simulink model "uas_demo"  (R2021a)
settings: Solver=FixedStepAuto  StartTime=0.0  StopTime=Inf  FixedStep=sample_time  RelTol=1e-3
model workspace: external: MAT-File (data not in the file)
values from neighbouring files (symbols this model uses):
  arm_length = 0.225    [Quadcopter_setup_parameters.m]    (also in recording.mat = 0.17; uas_parameters.m = 0.17; uas_parameters.mat = 0.17)
  drag_coefficient = 0.47    [Quadcopter_setup_parameters.m]    (also in recording.mat; uas_parameters.m; uas_parameters.mat)
  g = 9.81    [Quadcopter_setup_parameters.m]    (also in recording.mat = 9.80665; uas_parameters.m = 9.80665; uas_parameters.mat = 9.80665)
  inertia_xx = 5*10^(-3)    (= 0.005)    [Quadcopter_setup_parameters.m]    (also in recording.mat = 0.007; uas_parameters.m = 0.007; uas_parameters.mat = 0.007)
  inertia_yy = 5*10^(-3)    (= 0.005)    [Quadcopter_setup_parameters.m]    (also in recording.mat = 0.007; uas_parameters.m = 0.007; uas_parameters.mat = 0.007)
  inertia_zz = 8.9*10^(-3)    (= 0.0089)    [Quadcopter_setup_parameters.m]    (also in recording.mat = 0.012; uas_parameters.m = 0.012; uas_parameters.mat = 0.012)
  m = 0.55    [Quadcopter_setup_parameters.m]
  mass_drone = 0.55    [Quadcopter_setup_parameters.m]    (also in recording.mat = 0.68; uas_parameters.m = 0.68; uas_parameters.mat = 0.68)
  mass_total = mass_drone + mass_rod + mass_tip    (= 0.55)    [Quadcopter_setup_parameters.m]    (also in recording.mat = 0.68; uas_parameters.m = 0.68; uas_parameters.mat = 0.68)
  max_rot_velocity = 838    [Quadcopter_setup_parameters.m]    (also in recording.mat; uas_parameters.m; uas_parameters.mat)
  mix_matrix = inv(motor_constant * allocation_matrix)    [Quadcopter_setup_parameters.m]    (also in recording.mat = [29244.6230836 29244.6230836 29244.6230836 29244.6230836 -5.; uas_parameters.m; uas_parameters.mat = [29244.6230836 29244.6230836 29244.6230836 29244.6230836 -5.)
  moment_constant = 0.1    [Quadcopter_setup_parameters.m]    (also in recording.mat = 0.016; uas_parameters.m = 0.016; uas_parameters.mat = 0.016)
  motor_constant = 0.01    [Quadcopter_setup_parameters.m]    (also in recording.mat = 8.54858e-06; uas_parameters.m = 8.54858e-06; uas_parameters.mat = 8.54858e-06)
  p1 = 13.0908027334    [recording.mat]    (also in uas_parameters.mat = 12.1300541038; uas_thrust.mat = 12.1300541038; uas_thrust_constants.mat = 11.8019985126; uas_thrust_identification.m = result.p1)
  p2 = 0.438838137767    [recording.mat]    (also in uas_parameters.mat = 1.4832987942; uas_thrust.mat = 1.4832987942; uas_thrust_constants.mat = 1.1585190761; uas_thrust_identification.m = result.p2)
  poly_traj = PolyTrajGen(knots, order, optimization_target, dim, max_continuity)    [uas_minimum_snap.m]    (also in uas_trajectory.m = uas_minimum_snap(knots, order, waypoints, velocities, corrid)
  publish_rate = 1 * sample_time    (= 0.001)    [Quadcopter_setup_parameters.m]    (also in recording.mat = 0.04; uas_parameters.m = 0.04; uas_parameters.mat = 0.04)
  reference_area = pi * 75e-3^2    (= 0.0176714586764)    [Quadcopter_setup_parameters.m]    (also in recording.mat; uas_parameters.m; uas_parameters.mat)
  rotor_offset_top = 0.01    [Quadcopter_setup_parameters.m]    (also in recording.mat; uas_parameters.m; uas_parameters.mat)
  sample_time = 1e-3    (= 0.001)    [Quadcopter_setup_parameters.m]    (also in recording.mat = 0.04; uas_parameters.m = 0.04; uas_parameters.mat = 0.04)
  X = 3    [Quadcopter_setup_parameters.m]
  x0 = 36    [Quadcopter_setup_parameters.m]    (also in recording.mat; uas_parameters.m; uas_parameters.mat)
  Y = 2    [Quadcopter_setup_parameters.m]
  y0 = 80    [Quadcopter_setup_parameters.m]    (also in recording.mat; uas_parameters.m; uas_parameters.mat)
  Z = 1    [Quadcopter_setup_parameters.m]
  z0 = 1    [Quadcopter_setup_parameters.m]    (also in recording.mat = 0.3; uas_parameters.m; uas_parameters.mat)
undefined symbols (not defined in the file or in its folder): Angular, Linear, Pose, Position, Twist
libraries: nesl_utility x32, sm_lib x25, robotlib x13, simulink_extras x6, vrlib x1, sim3dlib x1, uavsim3dlib x1
(part 1 of 3)
settings Model: EnablePacing=on  Creator=david  LastModifiedBy=dwuth
settings SolverCC: AlgebraicLoopSolver=TrustRegion
settings DataIOCC: LimitDataPoints=on  MaxDataPoints=10000
settings OptimizationCC: EnhancedBackFolding=on  PassReuseOutputArgsThreshold=0  ZeroExternalMemoryAtStartup=off  ZeroInternalMemoryAtStartup=off  MaxStackSize=64  OptimizeBlockOrder=speed  DifferentSizesBufferReuse=on  OptimizationCustomize=off
settings DebuggingCC: ParameterTunabilityLossMsg=error  AllowSymbolicDim=off  SFUnexpectedBacktrackingDiag=warning  SFNoUnconditionalDefaultTransitionDiag=warning  SFExecutionAtInitializationDiag=none  SFMachineParentedDataDiag=warning  UnderSpecifiedDimensionMsg=warning  ArithmeticOperatorsInVariantConditions=warning
settings HardwareCC: ProdBitPerPointer=32  ProdBitPerSizeT=32  ProdBitPerPtrDiffT=32  ProdLargestAtomicFloat=None  ProdIntDivRoundTo=Undefined  ProdEndianess=Unspecified  ProdWordSize=32  ProdHWDeviceType=Generic->Unspecified (assume 32-bit Generic)  UseEmbeddedCoderFeatures=off
settings SFSimCC: SimUseLocalCustomCode=off  MATLABDynamicMemAlloc=off  CustomCodeUndefinedFunction=UseInterfaceOnly  SimTargetLang=C++
settings RTWCC: SystemTargetFile=ert.tlc  HardwareBoard=Robot Operating System (ROS)  TLCOptions="-aInlineSetEventsForThisBaseRateFcn=TLC_FALSE -aSuppressMultiTaskScheduler=TLC_FALSE  -aRateBasedStepFcn=0"  TemplateMakefile=ert_default_tmf  RTWUseLocalCustomCode=off  Toolchain=Catkin  TargetLang=C++
settings CodeAppCC: ForceParamTrailComments=on  OperatorAnnotations=on
settings ERTTargetCC: ERTCustomFileBanners=off  CodeInterfacePackaging=C++ class  SupportContinuousTime=on  SupportNonInlinedSFcns=on  RemoveResetFunc=off  ModelStepFunctionPrototypeControlCompliant=off  RootIOFormat=Structure reference
settings ConfigComp: CovMetricSettings=dw  CovSaveCumulativeToWorkspaceVar=on  CovSaveSingleToWorkspaceVar=on  CovExternalEMLEnable=off  CovSFcnEnable=off
settings SimscapeCC: SimscapeLogType=all  SimscapeLogSimulationStatistics=on  SimscapeLogDataHistory=10000

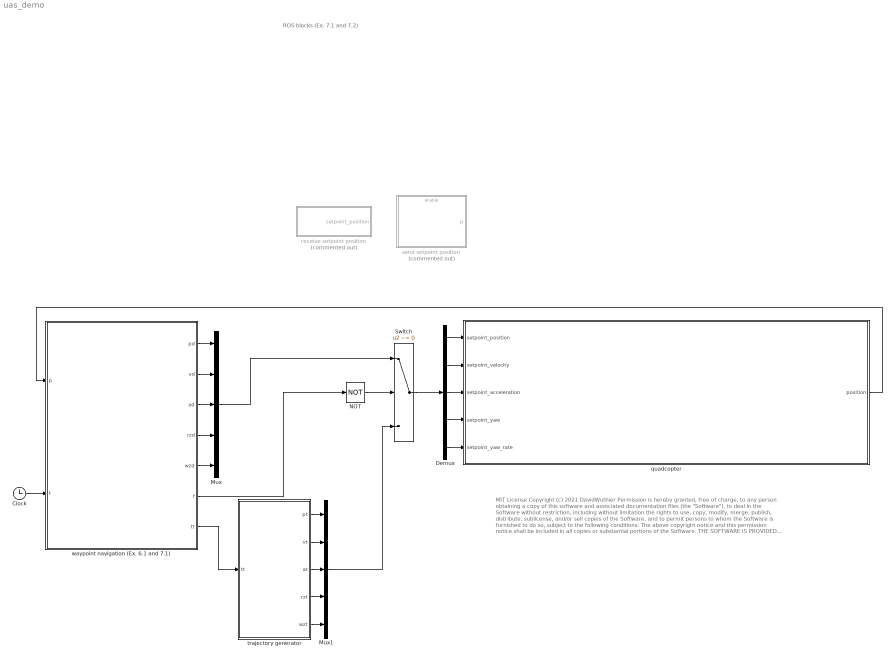
== system uas_demo ==
  note: MIT License
      |
      | Copyright (c) 2021 DavidWuthier
      |
      | Permission is hereby granted, free of charge, to any person obtaining a copy
      | of this software and associated documentation files (the "Software"), to deal
      | in the Software without restriction, including without limitation the rights
      | to use, copy, modify, merge, publish, distribute, sublicense, and/or sell
      | copies of the Software, and to permit persons to whom the Software is
      | furnished to do so, subject to the following conditions:
      |
      | The above copyright notice and this permission notice shall be included in all
      | copies or substantial portions of the Software.
      |
      | THE SOFTWARE IS PROVIDED "AS IS", WITHOUT WARRANTY OF ANY KIND, EXPRESS OR
      | IMPLIED, INCLUDING BUT NOT LIMITED TO THE WARRANTIES OF MERCHANTABILITY,
      | FITNESS FOR A PARTICULAR PURPOSE AND NONINFRINGEMENT. IN NO EVENT SHALL THE
      | AUTHORS OR COPYRIGHT HOLDERS BE LIABLE FOR ANY CLAIM, DAMAGES OR OTHER
      | LIABILITY, WHETHER IN AN ACTION OF CONTRACT, TORT OR OTHERWISE, ARISING FROM,
      | OUT OF OR IN CONNECTION WITH THE SOFTWARE OR THE USE OR OTHER DEALINGS IN THE
      | SOFTWARE.
  note: ROS blocks (Ex. 7.1 and 7.2)
  Clock : Clock
  Demux : Demux  Outputs=5
  Mux : Mux  Inputs=5
  Mux1 : Mux  Inputs=5
  NOT : Logic  Operator=NOT  IconShape=distinctive  AllPortsSameDT=off  OutDataTypeStr=boolean
  Switch : Switch  Criteria=u2 ~= 0
  quadcopter : Subsystem
  receive setpoint position : Subsystem  Commented=on
  send setpoint position : Subsystem  Commented=on
  trajectory generator : Subsystem
  waypoint navigation (Ex. 6.1 and 7.1) : Stateflow chart  TreatAsAtomicUnit=on
      settings: PortSchema="{\"entries\":[{\"content\":{\"sides\":[{\"content\":{\"connectorIds\":[\"In1\",\"In2\"]},\"type\":\"ConnectorPlacement.EquallySpacedRectSide\",\"uuid\":\"3b10aefc-58c0-4734-bcd6-9478d489aa11\"},{\"content\":{\"connectorIds\":[\"Out1\",\"Out2\",\"Out3\",\"Out7\",\"Out6\",\"Out5\",\"Out4\"],\"side\":\"RIGHT\"},\"type\":\"ConnectorPlacement.EquallySpacedRectSide\",\"uuid\":\"fcf7fbd2-2f8c-4d05-86e1-5a044196634d\"},{\"content\":{\"connectorIds\":[],\"side\":\"TOP\"},\"type\":\"ConnectorPlacement.EquallySpacedRectSide\",\"uuid\":\"94fc0c13-eb3b-4891-bff0-a1ef82a08378\"}]},\"type\":\"ConnectorPlacement.EquallySpacedConnector\",\"uuid\":\"15f9a3a1-5066-48dd-8188-11a3e0ea8b37\"}],\"packageUris\":[\"http://schema.mathworks.com/mf0/Connector/R2020b\"],\"version\":\"1.0\"}"
  wires:
  Clock/1 -> waypoint navigation (Ex. 6.1 and 7.1)/2(t)
  waypoint navigation (Ex. 6.1 and 7.1)/1(pd) -> Mux/1
  waypoint navigation (Ex. 6.1 and 7.1)/2(vd) -> Mux/2
  waypoint navigation (Ex. 6.1 and 7.1)/3(ad) -> Mux/3
  trajectory generator/1(pt) -> Mux1/1
  trajectory generator/2(vt) -> Mux1/2
  trajectory generator/3(at) -> Mux1/3
  waypoint navigation (Ex. 6.1 and 7.1)/4(tt) -> trajectory generator/1(tt)
  NOT/1 -> Switch/2
  waypoint navigation (Ex. 6.1 and 7.1)/5(f) -> NOT/1
  Mux1/1 -> Switch/3
  Mux/1 -> Switch/1
  Demux/1 -> quadcopter/1(setpoint_position)
  Demux/2 -> quadcopter/2(setpoint_velocity)
  Demux/3 -> quadcopter/3(setpoint_acceleration)
  Switch/1 -> Demux/1
  waypoint navigation (Ex. 6.1 and 7.1)/7(rzd) -> Mux/4
  waypoint navigation (Ex. 6.1 and 7.1)/6(wzd) -> Mux/5
  trajectory generator/4(rzt) -> Mux1/4
  trajectory generator/5(wzt) -> Mux1/5
  Demux/4 -> quadcopter/4(setpoint_yaw)
  Demux/5 -> quadcopter/5(setpoint_yaw_rate)
  quadcopter/1(position) -> waypoint navigation (Ex. 6.1 and 7.1)/1(p)

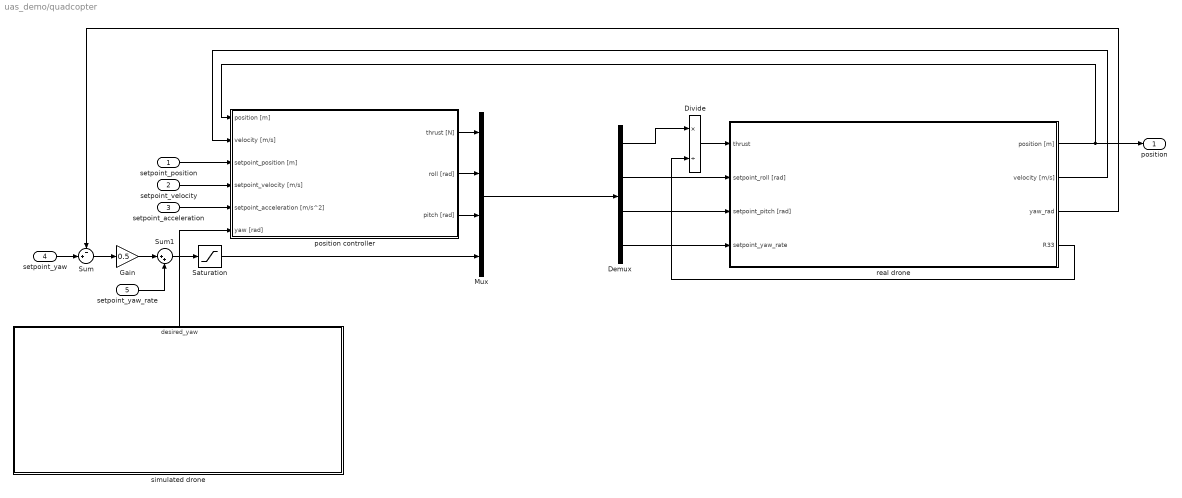
== system uas_demo/quadcopter ==
  setpoint_position : Inport  PortDimensions=[3 1]
  setpoint_velocity : Inport  Port=2  PortDimensions=[3 1]
  setpoint_acceleration : Inport  Port=3  PortDimensions=[3 1]
  setpoint_yaw : Inport  Port=4  PortDimensions=1
  setpoint_yaw_rate : Inport  Port=5  PortDimensions=1
  Demux : Demux
  Divide : Product  Inputs=*/
  Gain : Gain  Gain=0.5
  Mux : Mux
  Saturation : Saturate  UpperLimit=pi/2  LowerLimit=-pi/2
  Sum : Sum  Inputs=-+|
  Sum1 : Sum  Inputs=|++
  position controller : Subsystem
      mask Display: image('$imagefile'); % Use "Edit Image" on toolstrip to change.
  real drone : Subsystem
  simulated drone : Subsystem
      settings: PortSchema="{\"entries\":[{\"content\":{\"sides\":[{\"content\":{\"connectorIds\":[]},\"type\":\"ConnectorPlacement.EquallySpacedRectSide\",\"uuid\":\"a4b6e2c3-de70-4302-a56e-c646c409cb1c\"},{\"content\":{\"connectorIds\":[],\"side\":\"RIGHT\"},\"type\":\"ConnectorPlacement.EquallySpacedRectSide\",\"uuid\":\"cf331e27-abc1-4524-81a0-eea9b20dbeff\"},{\"content\":{\"connectorIds\":[\"Out1\"],\"side\":\"TOP\"},\"type\":\"ConnectorPlacement.EquallySpacedRectSide\",\"uuid\":\"8fd6f6ce-4f1c-4c94-a1c8-f1d72f1bbfd5\"},{\"content\":{\"connectorIds\":[],\"side\":\"BOTTOM\"},\"type\":\"ConnectorPlacement.EquallySpacedRectSide\",\"uuid\":\"db19f303-95c2-42a9-9683-bd7cccf66e90\"}]},\"type\":\"ConnectorPlacement.EquallySpacedConnector\",\"uuid\":\"27e9fd01-12c5-44cf-b1f4-f7b3cd5ad227\"}],\"packageUris\":[\"http://schema.mathworks.com/mf0/Connector/R2020b\"],\"version\":\"1.0\"}"
  position : Outport
  wires:
  setpoint_acceleration/1 -> position controller/5(setpoint_acceleration [m/s^2])
  setpoint_velocity/1 -> position controller/4(setpoint_velocity [m/s])
  setpoint_position/1 -> position controller/3(setpoint_position [m])
  position controller/1(thrust [N]) -> Mux/1
  position controller/2(roll [rad]) -> Mux/2
  position controller/3(pitch [rad]) -> Mux/3
  Demux/1 -> Divide/1
  Sum/1 -> Gain/1
  setpoint_yaw/1 -> Sum/2
  Gain/1 -> Sum1/1
  setpoint_yaw_rate/1 -> Sum1/2
  Sum1/1 -> Saturation/1
  Saturation/1 -> Mux/4
  real drone/1(position [m]) -> position/1, position controller/1(position [m])
  Divide/1 -> real drone/1(thrust)
  Demux/2 -> real drone/2(setpoint_roll [rad])
  Demux/3 -> real drone/3(setpoint_pitch [rad])
  Demux/4 -> real drone/4(setpoint_yaw_rate)
  real drone/2(velocity [m/s]) -> position controller/2(velocity [m/s])
  real drone/3(yaw_rad) -> Sum/1
  Mux/1 -> Demux/1
  simulated drone/1(desired_yaw) -> position controller/6(yaw [rad])
  real drone/4(R33) -> Divide/2

== system uas_demo/receive setpoint position ==
  Bus Selector : BusSelector  OutputSignals=Position.X,Position.Y,Position.Z
  Mux : Mux  Inputs=3
  Subscribe : robotlib/Subscribe  topicSource=Specify your own  topic=/crazyflie/cmd_position  messageType=geometry_msgs/Pose  SampleTime=-1  legacyBusStruct=off  messageQueueLength=1
  Terminator5 : Terminator
  setpoint_position : Outport
  wires:
  Subscribe/2 -> Bus Selector/1
  Mux/1 -> setpoint_position/1
  Bus Selector/3 -> Mux/3  "<Z>"
  Bus Selector/1 -> Mux/1  "<X>"
  Bus Selector/2 -> Mux/2  "<Y>"
  Subscribe/1 -> Terminator5/1

== system uas_demo/send setpoint position ==
  p : Inport
  Enable : EnablePort
  send setpoint position : Subsystem
  wires:
  p/1 -> send setpoint position/1(p)

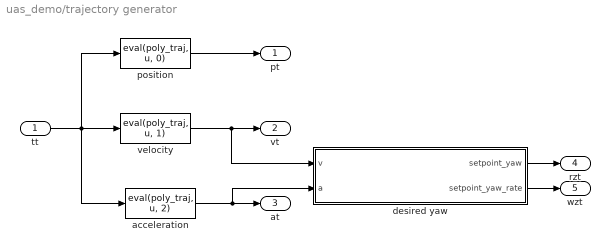
== system uas_demo/trajectory generator ==
  tt : Inport
  acceleration : MATLABFcn  MATLABFcn=eval(poly_traj, u, 2)  OutputDimensions=[3 1]  Output1D=off
  desired yaw : MATLAB Function  TreatAsAtomicUnit=on
  position : MATLABFcn  MATLABFcn=eval(poly_traj, u, 0)  OutputDimensions=[3 1]  Output1D=off
  velocity : MATLABFcn  MATLABFcn=eval(poly_traj, u, 1)  OutputDimensions=[3 1]  Output1D=off
  pt : Outport
  vt : Outport  Port=2
  at : Outport  Port=3
  rzt : Outport  Port=4
  wzt : Outport  Port=5
  wires:
  tt/1 -> acceleration/1, position/1, velocity/1
  velocity/1 -> desired yaw/1(v), vt/1
  position/1 -> pt/1
  acceleration/1 -> desired yaw/2(a), at/1
  desired yaw/1(setpoint_yaw) -> rzt/1
  desired yaw/2(setpoint_yaw_rate) -> wzt/1

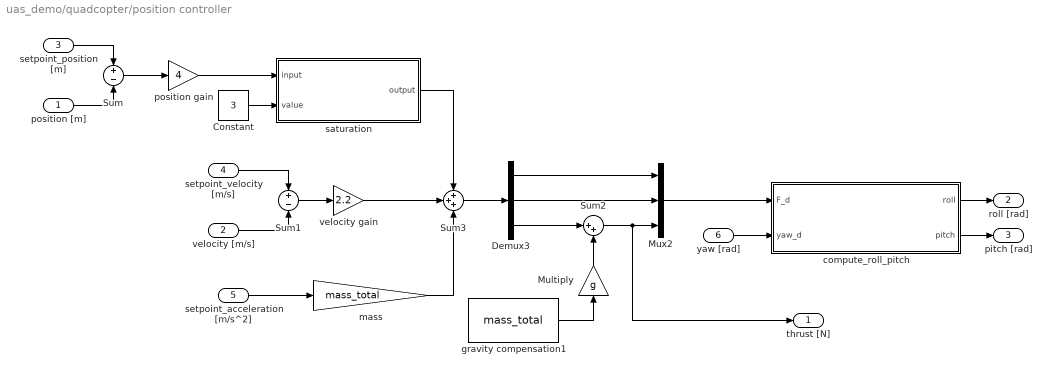
== system uas_demo/quadcopter/position controller ==
  position [m] : Inport
  velocity [m/s] : Inport  Port=2
  setpoint_position [m] : Inport  Port=3
  setpoint_velocity [m/s] : Inport  Port=4
  setpoint_acceleration [m/s^2] : Inport  Port=5
  yaw [rad] : Inport  Port=6
  Constant : Constant  Value=3
  Demux3 : Demux  Outputs=3
  Multiply : Gain  Gain=g
  Mux2 : Mux  Inputs=3
  Sum : Sum  Inputs=+|-
  Sum1 : Sum  Inputs=+|-
  Sum2 : Sum  Inputs=|++
  Sum3 : Sum  Inputs=+++
  compute_roll_pitch : MATLAB Function  TreatAsAtomicUnit=on
  gravity compensation1 : Constant  Value=mass_total  VectorParams1D=off
  mass : Gain  Gain=mass_total
  position gain : Gain  Gain=4
  saturation : Subsystem
  velocity gain : Gain  Gain=2.2
  thrust [N] : Outport
  roll [rad] : Outport  Port=2
  pitch [rad] : Outport  Port=3
  wires:
  saturation/1(output) -> Sum3/1
  position gain/1 -> saturation/1(input)
  gravity compensation1/1 -> Multiply/1
  velocity [m/s]/1 -> Sum1/2
  Demux3/3 -> Sum2/1
  mass/1 -> Sum3/3
  Constant/1 -> saturation/2(value)
  Sum2/1 -> thrust [N]/1, Mux2/3
  Sum1/1 -> velocity gain/1
  velocity gain/1 -> Sum3/2
  Sum/1 -> position gain/1
  Sum3/1 -> Demux3/1
  Demux3/1 -> Mux2/1
  Mux2/1 -> compute_roll_pitch/1(F_d)
  Demux3/2 -> Mux2/2
  compute_roll_pitch/1(roll) -> roll [rad]/1
  Multiply/1 -> Sum2/2
  setpoint_position [m]/1 -> Sum/1
  compute_roll_pitch/2(pitch) -> pitch [rad]/1
  position [m]/1 -> Sum/2
  yaw [rad]/1 -> compute_roll_pitch/2(yaw_d)
  setpoint_velocity [m/s]/1 -> Sum1/1
  setpoint_acceleration [m/s^2]/1 -> mass/1

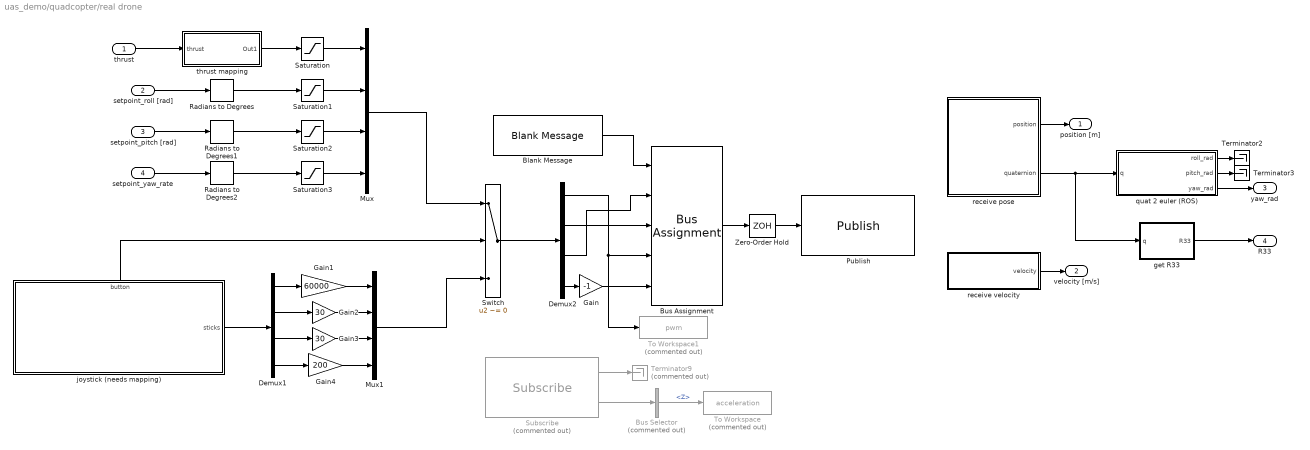
== system uas_demo/quadcopter/real drone ==
  thrust : Inport
  setpoint_roll [rad] : Inport  Port=2
  setpoint_pitch [rad] : Inport  Port=3
  setpoint_yaw_rate : Inport  Port=4
  Blank Message : robotlib/Blank Message  messageClass=Message  entityType=geometry_msgs/Twist  messageType=geometry_msgs/Twist  SampleTime=inf  legacyBusStruct=off
  Bus Assignment : BusAssignment  AssignedSignals=Linear.X,Linear.Y,Linear.Z,Angular.Z
  Bus Selector : BusSelector  Commented=on  OutputSignals=LinearAcceleration.Z
  Demux1 : Demux
  Demux2 : Demux
  Gain : Gain  Gain=-1
  Gain1 : Gain  Gain=60000
  Gain2 : Gain  Gain=30
  Gain3 : Gain  Gain=30
  Gain4 : Gain  Gain=200
  Mux : Mux
  Mux1 : Mux
  Publish : robotlib/Publish  topicSource=Select from ROS network  topic=/crazyflie/cmd_vel  messageType=geometry_msgs/Twist  legacyBusStruct=off  messageQueueLength=1
  Radians to Degrees : simulink_extras/Transformations/Radians to Degrees
  Radians to Degrees1 : simulink_extras/Transformations/Radians to Degrees
  Radians to Degrees2 : simulink_extras/Transformations/Radians to Degrees
  Saturation : Saturate  UpperLimit=50000  LowerLimit=5000
  Saturation1 : Saturate  UpperLimit=10  LowerLimit=-10
  Saturation2 : Saturate  UpperLimit=10  LowerLimit=-10
  Saturation3 : Saturate  UpperLimit=90  LowerLimit=-90
  Subscribe : robotlib/Subscribe  Commented=on  topicSource=Select from ROS network  topic=/crazyflie/imu  messageType=sensor_msgs/Imu  SampleTime=-1  legacyBusStruct=off  messageQueueLength=1
  Switch : Switch  Criteria=u2 ~= 0
  Terminator2 : Terminator
  Terminator3 : Terminator
  Terminator9 : Terminator  Commented=on
  To Workspace : ToWorkspace  Commented=on  VariableName=acceleration  SaveFormat=Timeseries  SampleTime=-1
  To Workspace1 : ToWorkspace  Commented=on  VariableName=pwm  SaveFormat=Timeseries  SampleTime=-1
  Zero-Order Hold : ZeroOrderHold  SampleTime=1/25
  get R33 : MATLAB Function  TreatAsAtomicUnit=on
  joystick (needs mapping) : Subsystem
      settings: PortSchema="{\"entries\":[{\"content\":{\"sides\":[{\"content\":{\"connectorIds\":[]},\"type\":\"ConnectorPlacement.EquallySpacedRectSide\",\"uuid\":\"5fda1310-e934-4f88-a5ae-12eb429239ff\"},{\"content\":{\"connectorIds\":[\"Out1\"],\"side\":\"RIGHT\"},\"type\":\"ConnectorPlacement.EquallySpacedRectSide\",\"uuid\":\"2a21e2c7-e332-4e9d-ba4f-bafdc6371a4a\"},{\"content\":{\"connectorIds\":[\"Out2\"],\"side\":\"TOP\"},\"type\":\"ConnectorPlacement.EquallySpacedRectSide\",\"uuid\":\"ad915a58-fa45-4be6-9ede-fc828b040a89\"}]},\"type\":\"ConnectorPlacement.EquallySpacedConnector\",\"uuid\":\"284bbdda-bb32-4fe9-aff6-c2c88357457c\"}],\"packageUris\":[\"http://schema.mathworks.com/mf0/Connector/R2020b\"],\"version\":\"1.0\"}"
  quat 2 euler (ROS) : MATLAB Function  TreatAsAtomicUnit=on
  receive pose : Subsystem
      settings: PortSchema="{\"entries\":[{\"content\":{\"sides\":[{\"content\":{\"connectorIds\":[\"Out1\",\"Out2\"]},\"type\":\"ConnectorPlacement.EquallySpacedRectSide\",\"uuid\":\"342eff32-bd5e-4bb8-a2c1-1476062da077\"},{\"content\":{\"connectorIds\":[],\"side\":\"RIGHT\"},\"type\":\"ConnectorPlacement.EquallySpacedRectSide\",\"uuid\":\"5f12c17c-6870-4adf-b6d3-8aed3aa982af\"},{\"content\":{\"connectorIds\":[],\"side\":\"TOP\"},\"type\":\"ConnectorPlacement.EquallySpacedRectSide\",\"uuid\":\"ee216cdd-c6bd-4d8d-9854-9a410974daca\"}]},\"type\":\"ConnectorPlacement.EquallySpacedConnector\",\"uuid\":\"aa6eedf3-0c3b-49f1-8a80-dfaeacb28973\"}],\"packageUris\":[\"http://schema.mathworks.com/mf0/Connector/R2020b\"],\"version\":\"1.0\"}"
  receive velocity : Subsystem
      settings: PortSchema="{\"entries\":[{\"content\":{\"sides\":[{\"content\":{\"connectorIds\":[\"Out1\"]},\"type\":\"ConnectorPlacement.EquallySpacedRectSide\",\"uuid\":\"342eff32-bd5e-4bb8-a2c1-1476062da077\"},{\"content\":{\"connectorIds\":[],\"side\":\"RIGHT\"},\"type\":\"ConnectorPlacement.EquallySpacedRectSide\",\"uuid\":\"5f12c17c-6870-4adf-b6d3-8aed3aa982af\"},{\"content\":{\"connectorIds\":[],\"side\":\"TOP\"},\"type\":\"ConnectorPlacement.EquallySpacedRectSide\",\"uuid\":\"ee216cdd-c6bd-4d8d-9854-9a410974daca\"}]},\"type\":\"ConnectorPlacement.EquallySpacedConnector\",\"uuid\":\"aa6eedf3-0c3b-49f1-8a80-dfaeacb28973\"}],\"packageUris\":[\"http://schema.mathworks.com/mf0/Connector/R2020b\"],\"version\":\"1.0\"}"
  thrust mapping : Subsystem
  position [m] : Outport
  velocity [m/s] : Outport  Port=2
  yaw_rad : Outport  Port=3
  R33 : Outport  Port=4
  wires:
  quat 2 euler (ROS)/2(pitch_rad) -> Terminator3/1
  quat 2 euler (ROS)/3(yaw_rad) -> yaw_rad/1
  quat 2 euler (ROS)/1(roll_rad) -> Terminator2/1
  receive pose/1(position) -> position [m]/1
  receive velocity/1(velocity) -> velocity [m/s]/1
  receive pose/2(quaternion) -> get R33/1(q), quat 2 euler (ROS)/1(q)
  thrust/1 -> thrust mapping/1(thrust)
  setpoint_roll [rad]/1 -> Radians to Degrees/1
  setpoint_pitch [rad]/1 -> Radians to Degrees1/1
  setpoint_yaw_rate/1 -> Radians to Degrees2/1
  Zero-Order Hold/1 -> Publish/1
  Demux2/3 -> Bus Assignment/2
  Demux2/4 -> Gain/1
  Blank Message/1 -> Bus Assignment/1
  Bus Assignment/1 -> Zero-Order Hold/1
  Demux2/2 -> Bus Assignment/3
  Demux2/1 -> To Workspace1/1, Bus Assignment/4
  Radians to Degrees/1 -> Saturation1/1
  Radians to Degrees1/1 -> Saturation2/1
  Radians to Degrees2/1 -> Saturation3/1
  Saturation1/1 -> Mux/2
  Saturation2/1 -> Mux/3
  Saturation3/1 -> Mux/4
  Saturation/1 -> Mux/1
  Switch/1 -> Demux2/1
  Mux/1 -> Switch/1
  Gain3/1 -> Mux1/3
  Gain2/1 -> Mux1/2
  Demux1/2 -> Gain2/1
  Demux1/3 -> Gain3/1
  Demux1/4 -> Gain4/1
  Demux1/1 -> Gain1/1
  Gain4/1 -> Mux1/4
  Gain1/1 -> Mux1/1
  joystick (needs mapping)/1(sticks) -> Demux1/1
  Mux1/1 -> Switch/3
  joystick (needs mapping)/2(button) -> Switch/2
  Bus Selector/1 -> To Workspace/1  "<Z>"
  Subscribe/1 -> Terminator9/1
  Subscribe/2 -> Bus Selector/1
  thrust mapping/1(Out1) -> Saturation/1
  Gain/1 -> Bus Assignment/5
  get R33/1(R33) -> R33/1

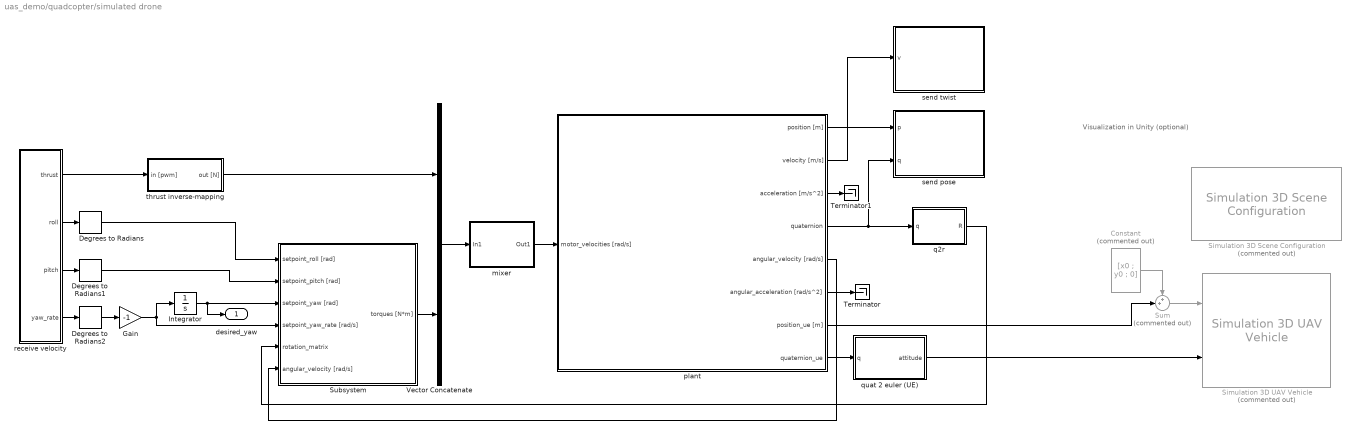
== system uas_demo/quadcopter/simulated drone ==
  note: Visualization in Unity (optional)
  Constant : Constant  Commented=on  Value=[x0 ; y0 ; 0]  VectorParams1D=off
  Degrees to Radians : simulink_extras/Transformations/Degrees to Radians
  Degrees to Radians1 : simulink_extras/Transformations/Degrees to Radians
  Degrees to Radians2 : simulink_extras/Transformations/Degrees to Radians
  Gain : Gain  Gain=-1
  Integrator : Integrator  WrapState=on
  Simulation 3D Scene Configuration : sim3dlib/Simulation 3D Scene Configuration  Priority=0  Commented=on  ProjectFormat=Default Scenes  SceneDesc=US city block  ProjectName=C:\Program Files\MATLAB\R2021a\toolbox\shared\sim3d_projects\automotive_project\UE4\WindowsNoEditor\VehicleSimulation.exe  ScenePath=/Game/Maps/USCityBlock  vehTagList={'Scene Origin';'SimulinkVehicle1'}  vehTag=SimulinkVehicle1  OpVisEn=off  Ts=sample_time  EnableWindow=on  EnableWeather=off  SunAltitude=40.0  SunAzimuth=90  clouds=10  wind=1  fog=0  rain=0  sensorTag=MainCamera1  sensorId=1  sensorName=MainCamera1  mountLoc=Origin  offsetFlag=off  tmountOffset=[0, 0, 0]  rmountOffset=[0, 0, 0]  HorizontalResolution=1280  VerticalResolution=720  HorizontalFOV=60  mountPoint=[0 0 0]  mountOrientation=[0 0 0]  aMode=4  ID=1
      settings: SourceProductBaseCode=DR,UV,VE
  Simulation 3D UAV Vehicle : uavsim3dlib/Simulation 3D UAV Vehicle  Commented=on  Mesh=Quadrotor  Color=Green  ActorName=SimulinkVehicle1  InitialTranslation=[x0 y0 z0]  InitialRotation=[0 0 0]  SampleTime=-1  ActorType=SimulinkVehicle  ID=1  aMode=4  ActorTag=SimulinkVehicle1
      settings: SourceProductBaseCode=UV
  Subsystem : Subsystem
      mask Display: image('$imagefile'); % Use "Edit Image" on toolstrip to change.
  Sum : Sum  Commented=on  Inputs=++|
  Terminator : Terminator
  Terminator1 : Terminator
  Vector Concatenate : Concatenate
  mixer : Subsystem
  plant : Subsystem
      mask Display: image('$imagefile'); % Use "Edit Image" on toolstrip to change.
  q2r : MATLAB Function  TreatAsAtomicUnit=on
  quat 2 euler (UE) : MATLAB Function  TreatAsAtomicUnit=on
  receive velocity : Subsystem
      settings: PortSchema="{\"entries\":[{\"content\":{\"sides\":[{\"content\":{\"connectorIds\":[\"Out1\",\"Out2\",\"Out3\",\"Out4\"]},\"type\":\"ConnectorPlacement.EquallySpacedRectSide\",\"uuid\":\"342eff32-bd5e-4bb8-a2c1-1476062da077\"},{\"content\":{\"connectorIds\":[],\"side\":\"RIGHT\"},\"type\":\"ConnectorPlacement.EquallySpacedRectSide\",\"uuid\":\"5f12c17c-6870-4adf-b6d3-8aed3aa982af\"},{\"content\":{\"connectorIds\":[],\"side\":\"TOP\"},\"type\":\"ConnectorPlacement.EquallySpacedRectSide\",\"uuid\":\"ee216cdd-c6bd-4d8d-9854-9a410974daca\"}]},\"type\":\"ConnectorPlacement.EquallySpacedConnector\",\"uuid\":\"aa6eedf3-0c3b-49f1-8a80-dfaeacb28973\"}],\"packageUris\":[\"http://schema.mathworks.com/mf0/Connector/R2020b\"],\"version\":\"1.0\"}"
  send pose : Subsystem
      settings: PortSchema="{\"entries\":[{\"content\":{\"sides\":[{\"content\":{\"connectorIds\":[]},\"type\":\"ConnectorPlacement.EquallySpacedRectSide\",\"uuid\":\"91ac49ce-0d45-467e-8a0f-3e047764dac5\"},{\"content\":{\"connectorIds\":[\"In1\",\"In2\"],\"side\":\"RIGHT\"},\"type\":\"ConnectorPlacement.EquallySpacedRectSide\",\"uuid\":\"1d243291-4bc7-414c-85ed-69dd8ac9cef1\"},{\"content\":{\"connectorIds\":[],\"side\":\"TOP\"},\"type\":\"ConnectorPlacement.EquallySpacedRectSide\",\"uuid\":\"579f94ca-36dc-4d39-8b83-523f53ee323c\"}]},\"type\":\"ConnectorPlacement.EquallySpacedConnector\",\"uuid\":\"95d78beb-d4cc-4232-87a4-7f0d7b157e3f\"}],\"packageUris\":[\"http://schema.mathworks.com/mf0/Connector/R2020b\"],\"version\":\"1.0\"}"
  send twist : Subsystem
      settings: PortSchema="{\"entries\":[{\"content\":{\"sides\":[{\"content\":{\"connectorIds\":[]},\"type\":\"ConnectorPlacement.EquallySpacedRectSide\",\"uuid\":\"91ac49ce-0d45-467e-8a0f-3e047764dac5\"},{\"content\":{\"connectorIds\":[\"In1\"],\"side\":\"RIGHT\"},\"type\":\"ConnectorPlacement.EquallySpacedRectSide\",\"uuid\":\"1d243291-4bc7-414c-85ed-69dd8ac9cef1\"},{\"content\":{\"connectorIds\":[],\"side\":\"TOP\"},\"type\":\"ConnectorPlacement.EquallySpacedRectSide\",\"uuid\":\"579f94ca-36dc-4d39-8b83-523f53ee323c\"}]},\"type\":\"ConnectorPlacement.EquallySpacedConnector\",\"uuid\":\"95d78beb-d4cc-4232-87a4-7f0d7b157e3f\"}],\"packageUris\":[\"http://schema.mathworks.com/mf0/Connector/R2020b\"],\"version\":\"1.0\"}"
  thrust inverse-mapping : Subsystem
  desired_yaw : Outport
  wires:
  quat 2 euler (UE)/1(attitude) -> Simulation 3D UAV Vehicle/2
  plant/5(angular_velocity [rad/s]) -> Subsystem/6(angular_velocity [rad/s])
  plant/3(acceleration [m/s^2]) -> Terminator1/1
  Vector Concatenate/1 -> mixer/1(In1)
  plant/6(angular_acceleration [rad/s^2]) -> Terminator/1
  q2r/1(R) -> Subsystem/5(rotation_matrix)
  mixer/1(Out1) -> plant/1(motor_velocities [rad/s])
  plant/8(quaternion_ue) -> quat 2 euler (UE)/1(q)
  Subsystem/1(torques [N*m]) -> Vector Concatenate/2
  Integrator/1 -> desired_yaw/1, Subsystem/3(setpoint_yaw [rad])
  plant/7(position_ue [m]) -> Sum/2
  receive velocity/4(yaw_rate) -> Degrees to Radians2/1
  receive velocity/2(roll) -> Degrees to Radians/1
  receive velocity/3(pitch) -> Degrees to Radians1/1
  Constant/1 -> Sum/1
  Sum/1 -> Simulation 3D UAV Vehicle/1
  plant/4(quaternion) -> send pose/2(q), q2r/1(q)
  plant/1(position [m]) -> send pose/1(p)
  plant/2(velocity [m/s]) -> send twist/1(v)
  Degrees to Radians/1 -> Subsystem/1(setpoint_roll [rad])
  Degrees to Radians1/1 -> Subsystem/2(setpoint_pitch [rad])
  Degrees to Radians2/1 -> Gain/1
  receive velocity/1(thrust) -> thrust inverse-mapping/1(in [pwm])
  thrust inverse-mapping/1(out [N]) -> Vector Concatenate/1
  Gain/1 -> Subsystem/4(setpoint_yaw_rate [rad/s]), Integrator/1

== system uas_demo/send setpoint position/send setpoint position ==
  p : Inport
  Blank Message : robotlib/Blank Message  messageClass=Message  entityType=geometry_msgs/Pose  messageType=geometry_msgs/Pose  SampleTime=inf  legacyBusStruct=off
  Bus Assignment : BusAssignment  AssignedSignals=Position.X,Position.Y,Position.Z
  Demux : Demux  Outputs=3
  Publish : robotlib/Publish  topicSource=Select from ROS network  topic=/crazyflie/cmd_position  messageType=geometry_msgs/Pose  legacyBusStruct=off  messageQueueLength=1
  Zero-Order Hold : ZeroOrderHold  SampleTime=publish_rate
  wires:
  Bus Assignment/1 -> Zero-Order Hold/1
  Blank Message/1 -> Bus Assignment/1
  Zero-Order Hold/1 -> Publish/1
  Demux/1 -> Bus Assignment/2
  Demux/2 -> Bus Assignment/3
  Demux/3 -> Bus Assignment/4
  p/1 -> Demux/1

== system uas_demo/quadcopter/position controller/saturation ==
  input : Inport
  value : Inport  Port=2
  Divide : Product  Inputs=**/
  Dot Product : DotProduct  InputSameDT=on  OutDataTypeStr=Inherit: Inherit via internal rule
  Sqrt1 : Sqrt  SaturateOnIntegerOverflow=on
  Sum3 : Sum  Inputs=-+|
  Switch : Switch  Criteria=u2 > Threshold
  output : Outport
  wires:
  Divide/1 -> Switch/1
  value/1 -> Divide/1, Sum3/1
  Dot Product/1 -> Sqrt1/1
  Switch/1 -> output/1
  Sum3/1 -> Switch/2
  input/1 -> Switch/3, Dot Product/2, Divide/2, Dot Product/1
  Sqrt1/1 -> Sum3/2, Divide/3

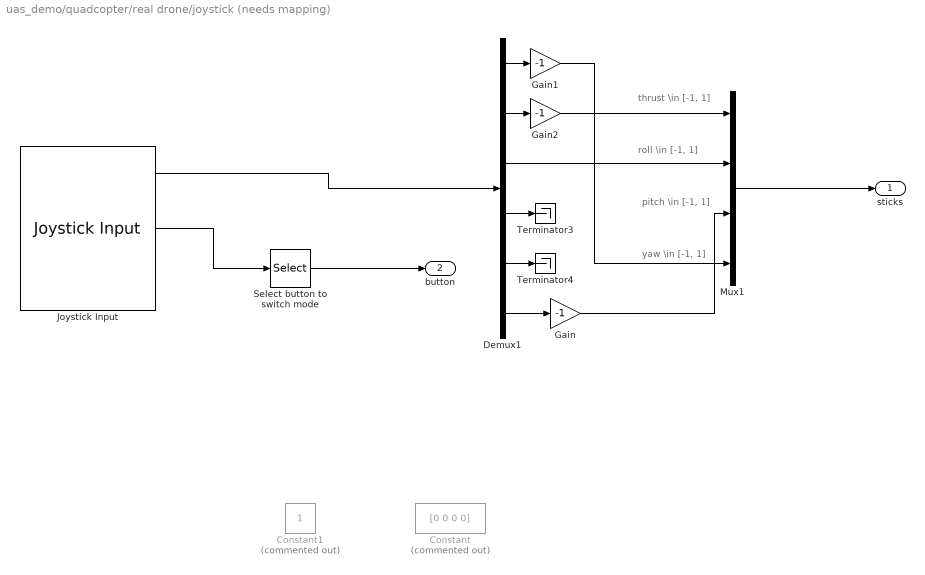
== system uas_demo/quadcopter/real drone/joystick (needs mapping) ==
  note: thrust \in [-1, 1]
  note: roll \in [-1, 1]
  note: pitch \in [-1, 1]
  note: yaw \in [-1, 1]
  Constant : Constant  Commented=on  Value=[0 0 0 0]
  Constant1 : Constant  Commented=on
  Demux1 : Demux  Outputs=6
  Gain : Gain  Gain=-1
  Gain1 : Gain  Gain=-1
  Gain2 : Gain  Gain=-1
  Joystick Input : vrlib/Joystick Input  joyid=1  adjustports=on  forcefeed=off
  Mux1 : Mux
  Select button to switch mode : Selector  InputPortWidth=15  IndexOptions=Index vector (dialog)  Indices=8  OutputSizes=1
  Terminator3 : Terminator
  Terminator4 : Terminator
  sticks : Outport
  button : Outport  Port=2
  wires:
  Gain1/1 -> Mux1/4
  Joystick Input/1 -> Demux1/1
  Gain2/1 -> Mux1/1
  Demux1/1 -> Gain1/1
  Joystick Input/2 -> Select button to switch mode/1
  Demux1/2 -> Gain2/1
  Gain/1 -> Mux1/3
  Select button to switch mode/1 -> button/1
  Mux1/1 -> sticks/1
  Demux1/4 -> Terminator3/1
  Demux1/6 -> Gain/1
  Demux1/3 -> Mux1/2
  Demux1/5 -> Terminator4/1

== system uas_demo/quadcopter/real drone/receive pose ==
  Bus Selector : BusSelector  OutputSignals=Pose.Position.X,Pose.Position.Y,Pose.Position.Z
  Bus Selector1 : BusSelector  OutputSignals=Pose.Orientation.W,Pose.Orientation.X,Pose.Orientation.Y,Pose.Orientation.Z
  Subscribe : robotlib/Subscribe  topicSource=Select from ROS network  topic=/crazyflie/pose  messageType=geometry_msgs/PoseStamped  SampleTime=-1  legacyBusStruct=off  messageQueueLength=1
  Terminator5 : Terminator
  Vector Concatenate : Concatenate  NumInputs=3  Mode=Multidimensional array
  Vector Concatenate1 : Concatenate  NumInputs=4  Mode=Multidimensional array  ConcatenateDimension=2
  position : Outport
  quaternion : Outport  Port=2
  wires:
  Subscribe/2 -> Bus Selector1/1, Bus Selector/1
  Vector Concatenate/1 -> position/1
  Bus Selector/3 -> Vector Concatenate/3  "<Z>"
  Bus Selector/1 -> Vector Concatenate/1  "<X>"
  Bus Selector/2 -> Vector Concatenate/2  "<Y>"
  Subscribe/1 -> Terminator5/1
  Bus Selector1/1 -> Vector Concatenate1/1  "<W>"
  Bus Selector1/2 -> Vector Concatenate1/2  "<X>"
  Bus Selector1/3 -> Vector Concatenate1/3  "<Y>"
  Vector Concatenate1/1 -> quaternion/1
  Bus Selector1/4 -> Vector Concatenate1/4  "<Z>"

== system uas_demo/quadcopter/real drone/receive velocity ==
  Bus Selector : BusSelector  OutputSignals=Twist.Linear.X,Twist.Linear.Y,Twist.Linear.Z
  Mux : Mux  Inputs=3
  Subscribe : robotlib/Subscribe  topicSource=Specify your own  topic=/crazyflie/twist  messageType=geometry_msgs/TwistStamped  SampleTime=-1  legacyBusStruct=off  messageQueueLength=1
  Terminator5 : Terminator
  velocity : Outport
  wires:
  Subscribe/2 -> Bus Selector/1
  Mux/1 -> velocity/1
  Bus Selector/3 -> Mux/3  "<Z>"
  Bus Selector/1 -> Mux/1  "<X>"
  Bus Selector/2 -> Mux/2  "<Y>"
  Subscribe/1 -> Terminator5/1

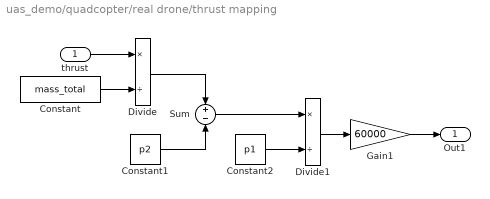
== system uas_demo/quadcopter/real drone/thrust mapping ==
  thrust : Inport
  Constant : Constant  Value=mass_total
  Constant1 : Constant  Value=p2
  Constant2 : Constant  Value=p1
  Divide : Product  Inputs=*/
  Divide1 : Product  Inputs=*/
  Gain1 : Gain  Gain=60000
  Sum : Sum  Inputs=+|-
  Out1 : Outport
  wires:
  thrust/1 -> Divide/1
  Constant/1 -> Divide/2
  Divide/1 -> Sum/1
  Constant1/1 -> Sum/2
  Sum/1 -> Divide1/1
  Constant2/1 -> Divide1/2
  Divide1/1 -> Gain1/1
  Gain1/1 -> Out1/1

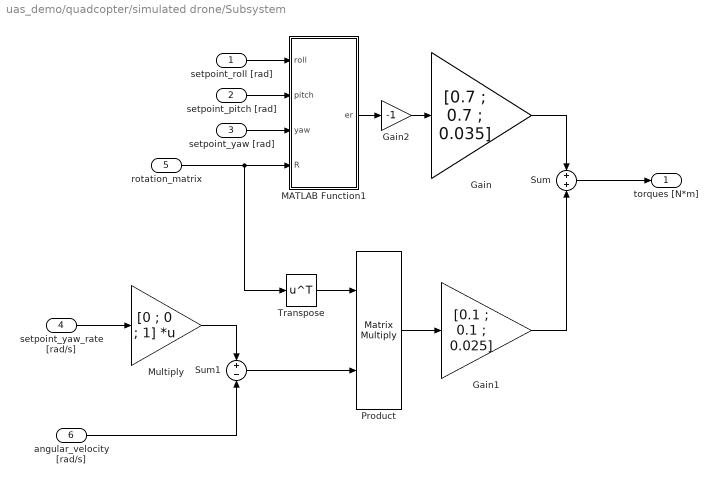
== system uas_demo/quadcopter/simulated drone/Subsystem ==
  setpoint_roll [rad] : Inport
  setpoint_pitch [rad] : Inport  Port=2
  setpoint_yaw [rad] : Inport  Port=3
  setpoint_yaw_rate [rad/s] : Inport  Port=4
  rotation_matrix : Inport  Port=5
  angular_velocity [rad/s] : Inport  Port=6
  Gain : Gain  Gain=[0.7 ; 0.7 ; 0.035]
  Gain1 : Gain  Gain=[0.1 ; 0.1 ; 0.025]
  Gain2 : Gain  Gain=-1
  MATLAB Function1 : MATLAB Function  TreatAsAtomicUnit=on
  Multiply : Gain  Gain=[0 ; 0 ; 1]  Multiplication=Matrix(K*u)
  Product : Product  Multiplication=Matrix(*)
  Sum : Sum
  Sum1 : Sum  Inputs=+|-
  Transpose : Math  Operator=transpose  SaturateOnIntegerOverflow=on
  torques [N*m] : Outport
  wires:
  rotation_matrix/1 -> Transpose/1, MATLAB Function1/4(R)
  setpoint_pitch [rad]/1 -> MATLAB Function1/2(pitch)
  Gain2/1 -> Gain/1
  Sum1/1 -> Product/2
  Gain1/1 -> Sum/2
  Multiply/1 -> Sum1/1
  Gain/1 -> Sum/1
  MATLAB Function1/1(er) -> Gain2/1
  setpoint_roll [rad]/1 -> MATLAB Function1/1(roll)
  setpoint_yaw [rad]/1 -> MATLAB Function1/3(yaw)
  Transpose/1 -> Product/1
  setpoint_yaw_rate [rad/s]/1 -> Multiply/1
  Product/1 -> Gain1/1
  angular_velocity [rad/s]/1 -> Sum1/2
  Sum/1 -> torques [N*m]/1

== system uas_demo/quadcopter/simulated drone/mixer ==
  In1 : Inport
  Gain5 : Gain  Gain=mix_matrix  Multiplication=Matrix(K*u)
  Saturation : Saturate  UpperLimit=max_rot_velocity^2  LowerLimit=0
  Sqrt : Sqrt  SaturateOnIntegerOverflow=on
  Out1 : Outport
  wires:
  Saturation/1 -> Sqrt/1
  In1/1 -> Gain5/1
  Sqrt/1 -> Out1/1
  Gain5/1 -> Saturation/1
